simulink model "p1_standalone"  (R2014a)
settings: Solver=ode1  SolverMode=SingleTasking  StartTime=0  StopTime=36000  FixedStep=Ts  RelTol=1e-3
PreLoadFcn:
  | InitModel
  | make
InitFcn:
  | InitModel
  | make
values from neighbouring files (symbols this model uses):
  num = num+MTnum(m)    [Build_MtMuMy.m]
  Ts = 0.002    [DSC_Control_Analysis.m]    (also in DSC_Control_Analysis_Exp.m; DSC_Speed_Control_Analysis.m; EC_params_nissan.m; Ext_MPCPara.m = SSD.Ts)
undefined symbols (not defined in the file or in its folder): den, DiscIntNeverNeededParam, gpsins, gr, hal_filter_den, hal_filter_num, Igain_l, Igain_r, Imax_l, Imax_r, Ioff_l, Ioff_r, KB, Kd, KF, Ki, KJ, Kp, param, sglu
libraries: simulink x5, slrtlib x3, xpcdiamondlib x2, UserBlocks x1
(part 3 of 3)

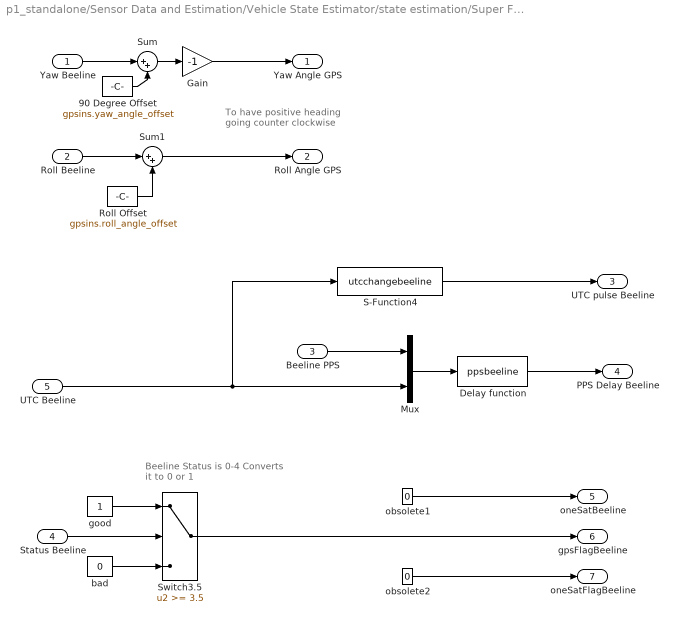
== system p1_standalone/Sensor Data and Estimation/Vehicle State Estimator/state estimation/Super Filter/Beeline GPS Pre-Processing ==
  note: Beeline Status is 0-4
      | Converts it to 0 or 1
  note: To have positive heading
      | going counter clockwise
  Yaw Beeline : Inport
  Roll Beeline : Inport  Port=2
  "Beeline PPS " : Inport  Port=3
  Status Beeline : Inport  Port=4
  UTC Beeline : Inport  Port=5
  90 Degree Offset : Constant  Value=gpsins.yaw_angle_offset
  Delay function : S-Function  FunctionName=ppsbeeline  Parameters=gpsins.maxbeelinedelay, Ts  EnableBusSupport=off
  Gain : Gain  Gain=-1  SaturateOnIntegerOverflow=on  OutDataTypeStr=Inherit: Same as input  ParamDataTypeStr=Inherit: Same as input
  Mux : Mux  Inputs=2
  Roll Offset : Constant  Value=gpsins.roll_angle_offset
  S-Function4 : S-Function  FunctionName=utcchangebeeline  Parameters=Ts  EnableBusSupport=off
  Sum : Sum  Inputs=|++  SaturateOnIntegerOverflow=on  InputSameDT=on  OutDataTypeStr=Inherit: Same as first input
  Sum1 : Sum  Inputs=|++  SaturateOnIntegerOverflow=on  InputSameDT=on  OutDataTypeStr=Inherit: Same as first input
  Switch3.5 : Switch  Threshold=3.5  SaturateOnIntegerOverflow=on  InputSameDT=on
  bad : Constant  Value=0
  good : Constant
  obsolete1 : Constant  Value=0
  obsolete2 : Constant  Value=0
  Yaw Angle GPS : Outport
  Roll Angle GPS : Outport  Port=2
  UTC pulse Beeline : Outport  Port=3
  PPS Delay Beeline : Outport  Port=4
  oneSatBeeline : Outport  Port=5
  gpsFlagBeeline : Outport  Port=6
  oneSatFlagBeeline : Outport  Port=7
  wires:
  Roll Offset/1 -> Sum1/2
  Sum1/1 -> Roll Angle GPS/1
  Roll Beeline/1 -> Sum1/1
  Yaw Beeline/1 -> Sum/1
  Sum/1 -> Gain/1
  90 Degree Offset/1 -> Sum/2
  Status Beeline/1 -> Switch3.5/2
  bad/1 -> Switch3.5/3
  good/1 -> Switch3.5/1
  S-Function4/1 -> UTC pulse Beeline/1
  Switch3.5/1 -> gpsFlagBeeline/1
  Delay function/1 -> PPS Delay Beeline/1
  "Beeline PPS "/1 -> Mux/1
  UTC Beeline/1 -> S-Function4/1, Mux/2
  Mux/1 -> Delay function/1
  obsolete2/1 -> oneSatFlagBeeline/1
  obsolete1/1 -> oneSatBeeline/1
  Gain/1 -> Yaw Angle GPS/1

== system p1_standalone/Sensor Data and Estimation/Vehicle State Estimator/state estimation/Super Filter/OEM4 GPS Pre-Processing ==
  OEM4 PPS : Inport
  UTC OEM4 : Inport  Port=2
  Vel status : Inport  Port=3
  Pos Status : Inport  Port=4
  Comparison to .1 : RelationalOperator  Operator===
  Constant : Constant  Value=.1
  Delay function : S-Function  FunctionName=ppsmillennium2  Parameters=gpsins.maxoem4delay, Ts  EnableBusSupport=off
  Mux : Mux  Inputs=2
  S-Function4 : S-Function  FunctionName=utcchangemillennium  Parameters=Ts  EnableBusSupport=off
  Sum : Sum  Inputs=|++  SaturateOnIntegerOverflow=on  InputSameDT=on  OutDataTypeStr=Inherit: Same as first input
  Switch : Switch  Threshold=2.5  SaturateOnIntegerOverflow=on  InputSameDT=on
  Switch1 : Switch  Threshold=3.5  SaturateOnIntegerOverflow=on  InputSameDT=on
  Switch2 : Switch  Threshold=1.5  SaturateOnIntegerOverflow=on  InputSameDT=on
  bad : Constant  Value=0
  bad1 : Constant  Value=0
  good : Constant
  good1 : Constant
  UTC Pulse OEM4 : Outport
  PPS Delay OEM4 : Outport  Port=2
  gpsFlagOEM4V : Outport  Port=3
  gpsFlagOEM4P : Outport  Port=4
  wires:
  UTC OEM4/1 -> S-Function4/1, Mux/2
  Switch2/1 -> gpsFlagOEM4V/1
  bad1/1 -> Switch2/3
  good1/1 -> Switch2/1
  Sum/1 -> Switch2/2
  Switch1/1 -> Sum/2
  Switch/1 -> Sum/1
  good/1 -> Switch1/3, Switch/1
  bad/1 -> Switch1/1, Switch/3
  Delay function/1 -> PPS Delay OEM4/1
  Mux/1 -> Delay function/1
  OEM4 PPS/1 -> Mux/1
  S-Function4/1 -> UTC Pulse OEM4/1
  Vel status/1 -> Switch/2, Switch1/2
  Constant/1 -> Comparison to .1/2
  Comparison to .1/1 -> gpsFlagOEM4P/1
  Pos Status/1 -> Comparison to .1/1

== system p1_standalone/Sensor Data and Estimation/Vehicle State Estimator/state estimation/Super Filter/Roll//Yaw Gyro Pre-processing ==
  Roll Gyro : Inport
  Yaw Gyro : Inport  Port=2
  Memory : Memory
  Roll Gyro Bias : Constant  Value=gpsins.roll_rate_bias
  Sum2 : Sum  Inputs=|++  SaturateOnIntegerOverflow=on  InputSameDT=on  OutDataTypeStr=Inherit: Same as first input
  Sum3 : Sum  Inputs=|+-  SaturateOnIntegerOverflow=on  InputSameDT=on  OutDataTypeStr=Inherit: Same as first input
  Sum4 : Sum  Inputs=|++  SaturateOnIntegerOverflow=on  InputSameDT=on  OutDataTypeStr=Inherit: Same as first input
  Sum5 : Sum  Inputs=|+-  SaturateOnIntegerOverflow=on  InputSameDT=on  OutDataTypeStr=Inherit: Same as first input
  Yaw Gyro Bias : Constant  Value=gpsins.yaw_rate_bias
  cross coupling from roll : Gain  Gain=gpsins.roll_to_yaw  SaturateOnIntegerOverflow=on  OutDataTypeStr=Inherit: Same as input  ParamDataTypeStr=Inherit: Same as input
  cross coupling from yaw : Gain  Gain=gpsins.yaw_to_roll  SaturateOnIntegerOverflow=on  OutDataTypeStr=Inherit: Same as input  ParamDataTypeStr=Inherit: Same as input
  roll rate sf : Gain  Gain=gpsins.roll_rate_sf  SaturateOnIntegerOverflow=on  OutDataTypeStr=Inherit: Same as input  ParamDataTypeStr=Inherit: Same as input
  yaw rate sf : Gain  SaturateOnIntegerOverflow=on  OutDataTypeStr=Inherit: Same as input  ParamDataTypeStr=Inherit: Same as input
  Yaw Rate : Outport
  Roll Rate : Outport  Port=2
  wires:
  Memory/1 -> cross coupling from roll/1
  Sum3/1 -> Memory/1, Roll Rate/1
  Sum5/1 -> cross coupling from yaw/1, Yaw Rate/1
  roll rate sf/1 -> Sum3/1
  yaw rate sf/1 -> Sum5/1
  cross coupling from roll/1 -> Sum5/2
  cross coupling from yaw/1 -> Sum3/2
  Sum4/1 -> roll rate sf/1
  Roll Gyro/1 -> Sum4/2
  Roll Gyro Bias/1 -> Sum4/1
  Yaw Gyro Bias/1 -> Sum2/2
  Sum2/1 -> yaw rate sf/1
  Yaw Gyro/1 -> Sum2/1

== system p1_standalone/Hardware I//O/Input/Handwheel Scaling & Initialization/Handwheel Sensor Fault Detection/Descision Logic/Change Detect ==
  1 : Inport
  2 : Inport  Port=2
  Abs : Abs
  Constant : Constant  Value=.1
  Relational Operator : RelationalOperator  Operator=>  OutDataTypeStr=float('double')
  Sum2 : Sum  Inputs=|+-
  Out : Outport
  wires:
  Sum2/1 -> Abs/1
  1/1 -> Sum2/1
  Abs/1 -> Relational Operator/1
  2/1 -> Sum2/2
  Relational Operator/1 -> Out/1
  Constant/1 -> Relational Operator/2

== system p1_standalone/Hardware I//O/Input/Handwheel Scaling & Initialization/Handwheel Sensor Fault Detection/Descision Logic/Latch ==
  Trigger : Inport
  Constant : Constant
  Enabled Subsystem : Subsystem  TreatAsAtomicUnit=on
  Triggered : Outport
  wires:
  Trigger/1 -> Enabled Subsystem/Enable
  Enabled Subsystem/1(Out1) -> Triggered/1
  Constant/1 -> Enabled Subsystem/1(In1)

== system p1_standalone/Hardware I//O/Input/Handwheel Scaling & Initialization/Handwheel Sensor Fault Detection/Descision Logic/Latch1 ==
  Trigger : Inport
  Constant : Constant
  Enabled Subsystem : Subsystem  TreatAsAtomicUnit=on
  Triggered : Outport
  wires:
  Trigger/1 -> Enabled Subsystem/Enable
  Enabled Subsystem/1(Out1) -> Triggered/1
  Constant/1 -> Enabled Subsystem/1(In1)

== system p1_standalone/Hardware I//O/Input/Handwheel Scaling & Initialization/Handwheel Sensor Fault Detection/Fault Detection1/Counter ==
  In : Inport
  Constant : Constant  Value=10
  Constant1 : Constant
  Discrete-Time Integrator : DiscreteIntegrator  ExternalReset=level  SampleTime=-1  LimitOutput=on  UpperSaturationLimit=10  LowerSaturationLimit=-10  ICPrevOutput=DiscIntNeverNeededParam  ICPrevScaledInput=DiscIntNeverNeededParam
  Relational Operator2 : RelationalOperator  Operator=>  OutDataTypeStr=float('double')
  Time : Outport
  wires:
  Relational Operator2/1 -> Time/1
  Constant1/1 -> Relational Operator2/2
  Discrete-Time Integrator/1 -> Relational Operator2/1
  Constant/1 -> Discrete-Time Integrator/1
  In/1 -> Discrete-Time Integrator/2

== system p1_standalone/Hardware I//O/Input/Handwheel Scaling & Initialization/Handwheel Sensor Fault Detection/Fault Detection1/Counter1 ==
  In : Inport
  Constant : Constant  Value=10
  Constant1 : Constant
  Discrete-Time Integrator : DiscreteIntegrator  ExternalReset=level  SampleTime=-1  LimitOutput=on  UpperSaturationLimit=10  LowerSaturationLimit=-10  ICPrevOutput=DiscIntNeverNeededParam  ICPrevScaledInput=DiscIntNeverNeededParam
  Relational Operator2 : RelationalOperator  Operator=>  OutDataTypeStr=float('double')
  Time : Outport
  wires:
  Relational Operator2/1 -> Time/1
  Constant1/1 -> Relational Operator2/2
  Discrete-Time Integrator/1 -> Relational Operator2/1
  Constant/1 -> Discrete-Time Integrator/1
  In/1 -> Discrete-Time Integrator/2

== system p1_standalone/Hardware I//O/Input/Handwheel Scaling & Initialization/Handwheel Sensor Fault Detection/Fault Detection1/Enabled Subsystem ==
  In1 : Inport
  Enable : EnablePort
  Out1 : Outport
  wires:
  In1/1 -> Out1/1

== system p1_standalone/Hardware I//O/Input/Handwheel Scaling & Initialization/Handwheel Sensor Fault Detection/Fault Detection1/Enabled Subsystem1 ==
  In1 : Inport
  Enable : EnablePort
  Out1 : Outport
  wires:
  In1/1 -> Out1/1

== system p1_standalone/Hardware I//O/Input/Handwheel Scaling & Initialization/Handwheel Sensor Fault Detection/Fault Detection1/Nearly the Same ==
  1 : Inport
  2 : Inport  Port=2
  Abs : Abs
  Constant : Constant  Value=.0001
  Relational Operator : RelationalOperator  Operator=>  OutDataTypeStr=float('double')
  Sum2 : Sum  Inputs=|+-
  Out : Outport
  wires:
  Constant/1 -> Relational Operator/2
  Relational Operator/1 -> Out/1
  2/1 -> Sum2/2
  Abs/1 -> Relational Operator/1
  1/1 -> Sum2/1
  Sum2/1 -> Abs/1

== system p1_standalone/Hardware I//O/Input/Handwheel Scaling & Initialization/Handwheel Sensor Fault Detection/Fault Detection1/Nearly the Same1 ==
  1 : Inport
  2 : Inport  Port=2
  Abs : Abs
  Constant : Constant  Value=.1
  Relational Operator : RelationalOperator  Operator=>  OutDataTypeStr=float('double')
  Sum2 : Sum  Inputs=|+-
  Out : Outport
  wires:
  Constant/1 -> Relational Operator/2
  Relational Operator/1 -> Out/1
  2/1 -> Sum2/2
  Abs/1 -> Relational Operator/1
  1/1 -> Sum2/1
  Sum2/1 -> Abs/1

== system p1_standalone/Hardware I//O/Input/Handwheel Scaling & Initialization/Handwheel Sensor Fault Detection/Fault Detection1/Nearly the Same2 ==
  1 : Inport
  2 : Inport  Port=2
  Abs : Abs
  Constant : Constant  Value=.0001
  Relational Operator : RelationalOperator  Operator=>  OutDataTypeStr=float('double')
  Sum2 : Sum  Inputs=|+-
  Out : Outport
  wires:
  Sum2/1 -> Abs/1
  1/1 -> Sum2/1
  Abs/1 -> Relational Operator/1
  2/1 -> Sum2/2
  Relational Operator/1 -> Out/1
  Constant/1 -> Relational Operator/2

== system p1_standalone/Hardware I//O/Input/Handwheel Scaling & Initialization/Handwheel Sensor Fault Detection/Fault Detection1/Nearly the Same3 ==
  1 : Inport
  2 : Inport  Port=2
  Abs : Abs
  Constant : Constant  Value=.2
  Relational Operator : RelationalOperator  Operator=>  OutDataTypeStr=float('double')
  Sum2 : Sum  Inputs=|+-
  Out : Outport
  wires:
  Sum2/1 -> Abs/1
  1/1 -> Sum2/1
  Abs/1 -> Relational Operator/1
  2/1 -> Sum2/2
  Relational Operator/1 -> Out/1
  Constant/1 -> Relational Operator/2

== system p1_standalone/Hardware I//O/Input/Handwheel Scaling & Initialization/Handwheel Sensor Fault Detection/Descision Logic/Latch/Enabled Subsystem ==
  In1 : Inport
  Enable : EnablePort
  Out1 : Outport
  wires:
  In1/1 -> Out1/1

== system p1_standalone/Hardware I//O/Input/Handwheel Scaling & Initialization/Handwheel Sensor Fault Detection/Descision Logic/Latch1/Enabled Subsystem ==
  In1 : Inport
  Enable : EnablePort
  Out1 : Outport
  wires:
  In1/1 -> Out1/1
